simulink model "model"  (R2023a)
settings: Solver=VariableStepAuto  StartTime=0.0  StopTime=tsim  RelTol=1e-3
values from neighbouring files (symbols this model uses):
  mu = 1    [main.m]
  x1_0 = 0.01    [main.m]
  x2_0 = 0.01    [main.m]
settings Model: Creator=eriknymobohne  LastModifiedBy=eriknymobohne

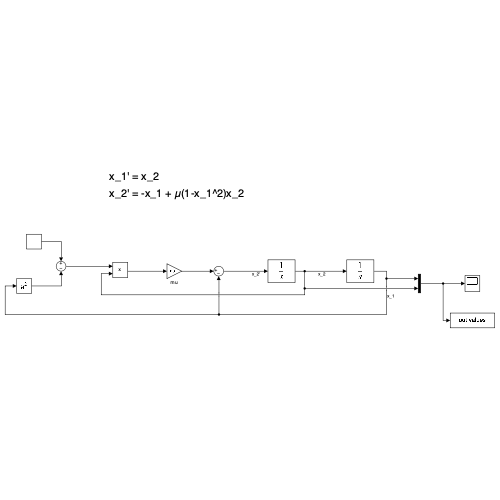
[thumbnail: Simulink's stored preview of the top-level diagram]
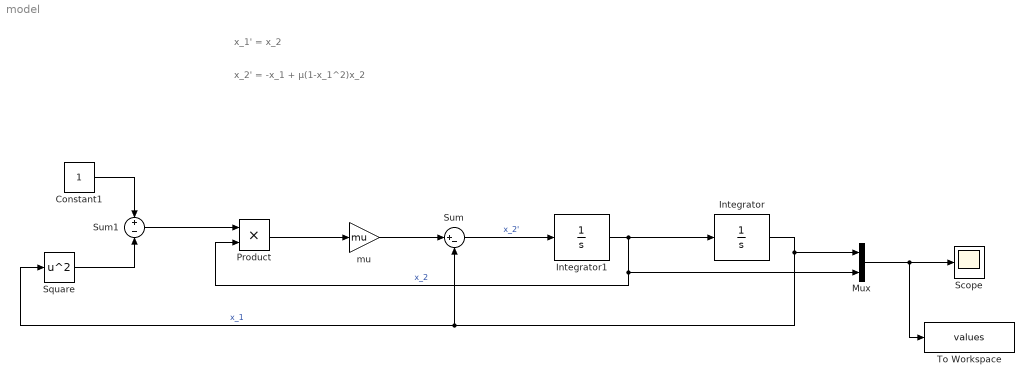
== system model ==
  note: x_1' = x_2
  note: x_2' = -x_1 + µ(1-x_1^2)x_2
  Constant1 : Constant
  Integrator : Integrator  InitialCondition=x1_0
  Integrator1 : Integrator  InitialCondition=x2_0
  Mux : Mux  Inputs=2
  Product : Product
  Scope : Scope
  Square : Math  Operator=square
  Sum : Sum  Inputs=|+-
  Sum1 : Sum  Inputs=+-
  To Workspace : ToWorkspace  VariableName=values  SaveFormat=Timeseries  SampleTime=-1
  mu : Gain  Gain=mu
  wires:
  Integrator1/1 -> Product/2, Mux/2, Integrator/1  "x_2"
  Integrator/1 -> Mux/1, Sum/2, Square/1  "x_1"
  Sum/1 -> Integrator1/1  "x_2'"
  mu/1 -> Sum/1
  Product/1 -> mu/1
  Square/1 -> Sum1/2
  Sum1/1 -> Product/1
  Constant1/1 -> Sum1/1
  Mux/1 -> To Workspace/1, Scope/1
